simulink model "toilet"  (Simulink 6.0)
settings: Solver=ode1  SolverMode=SingleTasking  StartTime=0.0  StopTime=inf  FixedStep=.5  RelTol=1e-3  AbsTol=1e-6
PreLoadFcn:
  | toiletgui
StartFcn:
  | toiletgui start
StopFcn:
  | toiletgui stop
values from neighbouring files (symbols this model uses):
  area = 100    [toiletgui.m]
  hilim = evalin('base','hilim')    [toiletgui.m]
  inflow = 10    [toiletgui.m]
  lolim = evalin('base','lolim')    [toiletgui.m]
  outflow = 50    [toiletgui.m]
CloseFcn:
  | toiletgui done
settings Model: Creator=The MathWorks Inc.  LastModifiedBy=batserve  ExtModeTrigMode=oneshot  ExtModeArmWhenConnect=off  ExtModeAutoUpdateStatusClock=off
settings DataIOCC: LimitDataPoints=off
settings DebuggingCC: CheckExecutionContextPreStartOutputMsg=on  CheckExecutionContextRuntimeOutputMsg=on  SolverPrmCheckMsg=none  IntegerOverflowMsg=none
settings HardwareCC: TargetUnknown=on

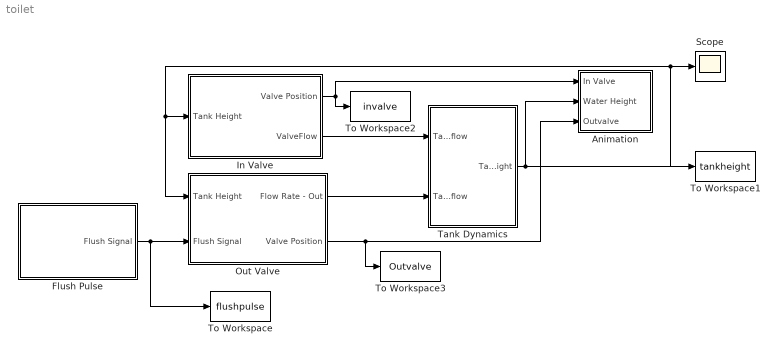
== system toilet ==
  Animation : Subsystem  PropExecContextAcrossSSBoundary=on
      mask Display: disp('Animation\nControl')
  Flush Pulse : Subsystem  PropExecContextAcrossSSBoundary=on
      settings: OpenFcn=toiletgui flush
      mask Display: disp('Double Click\nTo\nFlush Me!')
  In Valve : Subsystem  PropExecContextAcrossSSBoundary=on  mask{hilim=hilim, inflow=inflow}
      mask prompts: hilim "Shut Off Height"; inflow "Flow Rate"
  Out Valve : Subsystem  PropExecContextAcrossSSBoundary=on
  Scope : Scope
      settings: TickLabels=on  TimeRange=20  YMin=0  YMax=12.5  DataFormat=Array
  Tank Dynamics : Subsystem  PropExecContextAcrossSSBoundary=on
  To Workspace : ToWorkspace  VariableName=flushpulse  SampleTime=-1  SaveFormat=Array
  To Workspace1 : ToWorkspace  VariableName=tankheight  SampleTime=-1  SaveFormat=Array
  To Workspace2 : ToWorkspace  VariableName=invalve  SampleTime=-1  SaveFormat=Array
  To Workspace3 : ToWorkspace  VariableName=Outvalve  SampleTime=-1  SaveFormat=Array
  wires:
  Out Valve/2(Valve Position) -> Animation/3(Outvalve), To Workspace3/1
  In Valve/1(Valve Position) -> Animation/1(In Valve), To Workspace2/1
  Tank Dynamics/1(Tank Height) -> Scope/1, Out Valve/1(Tank Height), In Valve/1(Tank Height), Animation/2(Water Height), To Workspace1/1
  In Valve/2(ValveFlow) -> Tank Dynamics/1(Tank Inflow)
  Flush Pulse/1(Flush Signal) -> Out Valve/2(Flush Signal), To Workspace/1
  Out Valve/1(Flow Rate - Out) -> Tank Dynamics/2(Tank Outflow)

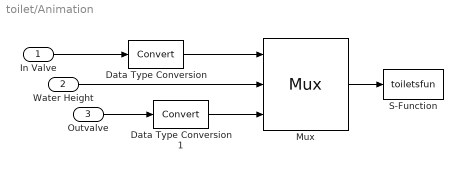
== system toilet/Animation ==
  In Valve : Inport  Port=1  LatchInput=off
  Water Height : Inport  Port=2  LatchInput=off
  Outvalve : Inport  Port=3  LatchInput=off
  Data Type Conversion : DataTypeConversion  OutDataTypeMode=double  SaturateOnIntegerOverflow=on  RndMeth=Zero
  Data Type Conversion1 : DataTypeConversion  OutDataTypeMode=double  SaturateOnIntegerOverflow=on  RndMeth=Zero
  Mux : Mux  Inputs=3
  S-Function : S-Function  FunctionName=toiletsfun  Parameters=inflow,outflow,lolim,hilim,area
  wires:
  Outvalve/1 -> Data Type Conversion1/1
  Water Height/1 -> Mux/2
  Mux/1 -> S-Function/1
  In Valve/1 -> Data Type Conversion/1
  Data Type Conversion1/1 -> Mux/3
  Data Type Conversion/1 -> Mux/1

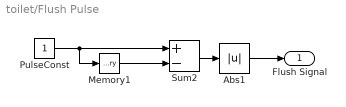
== system toilet/Flush Pulse ==
  Abs1 : Abs  SaturateOnIntegerOverflow=on
  Memory1 : Memory
  PulseConst : Constant
  Sum2 : Sum  Inputs=+-  SaturateOnIntegerOverflow=on  InputSameDT=on
  Flush Signal : Outport  InitialOutput=0
  wires:
  PulseConst/1 -> Sum2/1, Memory1/1
  Sum2/1 -> Abs1/1
  Memory1/1 -> Sum2/2
  Abs1/1 -> Flush Signal/1

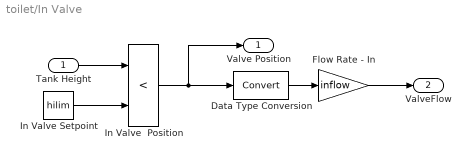
== system toilet/In Valve ==
  Tank Height : Inport  Port=1  LatchInput=off
  Data Type Conversion : DataTypeConversion  OutDataTypeMode=double  SaturateOnIntegerOverflow=on  RndMeth=Zero
  Flow Rate - In : Gain  Gain=inflow  SaturateOnIntegerOverflow=on
  In Valve  Position : RelationalOperator  Operator=<  InputSameDT=on
  In Valve Setpoint : Constant  Value=hilim
  Valve Position : Outport  InitialOutput=0
  ValveFlow : Outport  Port=2  InitialOutput=0
  wires:
  Flow Rate - In/1 -> ValveFlow/1
  In Valve  Position/1 -> Valve Position/1, Data Type Conversion/1
  Tank Height/1 -> In Valve  Position/1
  In Valve Setpoint/1 -> In Valve  Position/2
  Data Type Conversion/1 -> Flow Rate - In/1

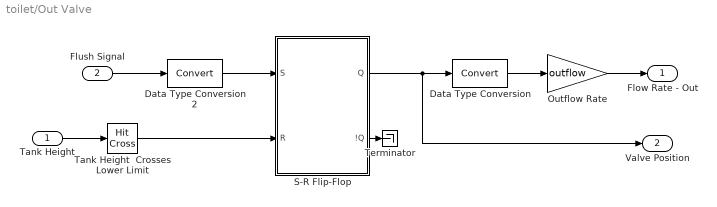
== system toilet/Out Valve ==
  Tank Height : Inport  Port=1  LatchInput=off
  Flush Signal : Inport  Port=2  LatchInput=off
  Data Type Conversion : DataTypeConversion  OutDataTypeMode=double  SaturateOnIntegerOverflow=on  RndMeth=Zero
  Data Type Conversion2 : DataTypeConversion  OutDataTypeMode=boolean  SaturateOnIntegerOverflow=on  RndMeth=Zero
  Outflow Rate : Gain  Gain=outflow  SaturateOnIntegerOverflow=on
  S-R Flip-Flop : Subsystem  PropExecContextAcrossSSBoundary=on
      mask Type: S-R Flip-Flop
  Tank Height  Crosses Lower Limit : HitCross  HitCrossingOffset=lolim  HitCrossingDirection=falling
  Terminator : Terminator
  Flow Rate - Out : Outport  InitialOutput=0
  Valve Position : Outport  Port=2  InitialOutput=0
  wires:
  Tank Height/1 -> Tank Height  Crosses Lower Limit/1
  Tank Height  Crosses Lower Limit/1 -> S-R Flip-Flop/2(R)
  S-R Flip-Flop/1(Q) -> Valve Position/1, Data Type Conversion/1
  Flush Signal/1 -> Data Type Conversion2/1
  S-R Flip-Flop/2(!Q) -> Terminator/1
  Outflow Rate/1 -> Flow Rate - Out/1
  Data Type Conversion/1 -> Outflow Rate/1
  Data Type Conversion2/1 -> S-R Flip-Flop/1(S)

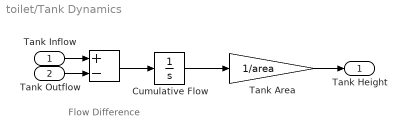
== system toilet/Tank Dynamics ==
  note: Flow
      | Difference
  Tank Inflow : Inport  Port=1  LatchInput=off
  Tank Outflow : Inport  Port=2  LatchInput=off
  " " : Sum  Inputs=+-  SaturateOnIntegerOverflow=on  InputSameDT=on
  Cumulative Flow : Integrator  InitialCondition=(hilim+lolim)/2*area
  Tank Area : Gain  Gain=1/area  SaturateOnIntegerOverflow=on
  Tank Height : Outport  InitialOutput=0
  wires:
  Tank Outflow/1 -> " "/2
  Tank Inflow/1 -> " "/1
  " "/1 -> Cumulative Flow/1
  Cumulative Flow/1 -> Tank Area/1
  Tank Area/1 -> Tank Height/1

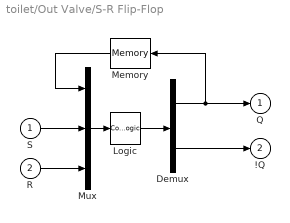
== system toilet/Out Valve/S-R Flip-Flop ==
  S : Inport  Port=1  LatchInput=off
  R : Inport  Port=2  LatchInput=off
  Demux : Demux  Outputs=2
  Logic : CombinatorialLogic  TruthTable=[0 1;0 1;1 0;0 1;1 0;0 1;1 0;1 0]
  Memory : Memory  Orientation=left  InheritSampleTime=on
  Mux : Mux  Inputs=3
  Q : Outport  InitialOutput=0
  !Q : Outport  Port=2  InitialOutput=1
  wires:
  R/1 -> Mux/3
  S/1 -> Mux/2
  Memory/1 -> Mux/1
  Demux/1 -> Memory/1, Q/1
  Demux/2 -> !Q/1
  Logic/1 -> Demux/1
  Mux/1 -> Logic/1
